simulink subsystem "PIDAntiWindupDigital_SubSystem"  (R2020b)
settings: Solver=VariableStepAuto  StartTime=0.0  StopTime=10.0  RelTol=1e-3
values from neighbouring files (symbols this model uses):
  CDer = CBEDer    [PIDAntiWindupDigital.m]    (also in PIDDigital.m = CTustinDer)
  CInt = CBEInt    [PIDAntiWindupDigital.m]    (also in PIDDigital.m = CTustinInt)
  Kd = 0    [PIDesigner.m]    (also in loadParamExperiment.m = 0.2578)
  Ki = -wgc*deltaK*sin(deltaPhm)    [PIDesigner.m]    (also in loadParamExperiment.m = 1.1459)
  Kp = deltaK*cos(deltaPhm)    [PIDesigner.m]    (also in loadParamExperiment.m = 37.8152)
  Kw = 1/Tw    (= 33.3333333333)    [PIDAntiWindupDigital.m]
  Ts = T2    (= 0.01)    [PIDAntiWindupDigital.m]    (also in PIDDigital.m = 0.001; StateSpaceControllerNominalCont.m = 0.001; StateSpaceControllerNominalDigital.m = 0.001; StateSpaceControllerNominalDirectDigital.m = 0.05)
settings Model: Creator=umbe  LastModifiedBy=umbe

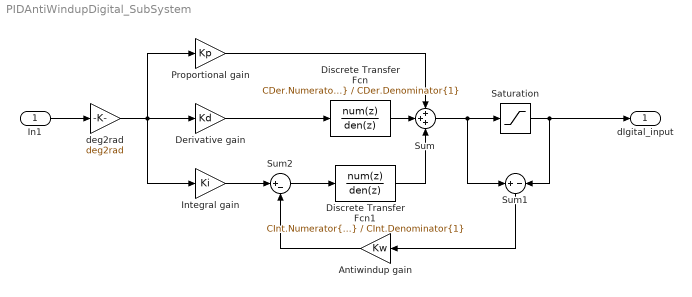
== system PIDAntiWindupDigital_SubSystem ==
  In1 : Inport
  Antiwindup gain : Gain  Gain=Kw
  Derivative gain : Gain  Gain=Kd
  Discrete Transfer Fcn : DiscreteTransferFcn  Numerator=CDer.Numerator{1}  Denominator=CDer.Denominator{1}  SampleTime=Ts
  Discrete Transfer Fcn1 : DiscreteTransferFcn  Numerator=CInt.Numerator{1}  Denominator=CInt.Denominator{1}  SampleTime=Ts
  Integral gain : Gain  Gain=Ki
  Proportional gain : Gain  Gain=Kp
  Saturation : Saturate  UpperLimit=10  LowerLimit=-10
  Sum : Sum  Inputs=+++
  Sum1 : Sum  Inputs=+|-
  Sum2 : Sum  Inputs=|+-
  deg2rad : Gain  Gain=deg2rad
  dIgital_input : Outport
  wires:
  Proportional gain/1 -> Sum/1
  Discrete Transfer Fcn/1 -> Sum/2
  Derivative gain/1 -> Discrete Transfer Fcn/1
  Discrete Transfer Fcn1/1 -> Sum/3
  deg2rad/1 -> Integral gain/1, Derivative gain/1, Proportional gain/1
  In1/1 -> deg2rad/1
  Antiwindup gain/1 -> Sum2/2
  Sum1/1 -> Antiwindup gain/1
  Saturation/1 -> dIgital_input/1, Sum1/2
  Sum/1 -> Sum1/1, Saturation/1
  Integral gain/1 -> Sum2/1
  Sum2/1 -> Discrete Transfer Fcn1/1
